simulink subsystem "DYNAMICS"  (R2025b)
settings: Solver=VariableStepAuto  StartTime=0.0  StopTime=10.0  RelTol=1e-3
settings Model: Creator=antoniohernandez-rodiciomateos  LastModifiedBy=antoniohernandez-rodiciomateos

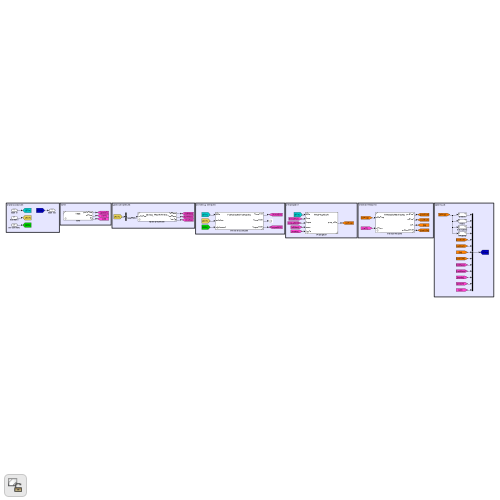
[thumbnail: Simulink's stored preview of the top-level diagram]
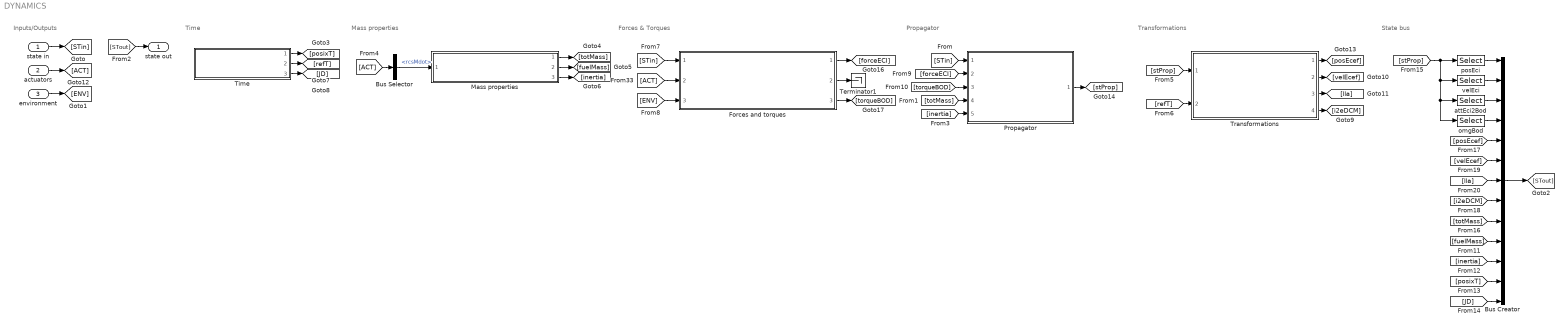
== system DYNAMICS ==
  note: Inputs/Outputs
  note: Mass properties
  note: Time
  note: Forces & Torques
  note: Propagator
  note: Transformations
  note: State bus
  state in : Inport  OutDataTypeStr=Bus: state_bus
  actuators : Inport  Port=2
  environment : Inport  Port=3  OutDataTypeStr=Bus: environment_bus
  Bus Creator : BusCreator  Inputs=13  OutDataTypeStr=Bus: state_bus  NonVirtualBus=on
      settings: InheritFromInputs=off
  Bus Selector : BusSelector  OutputSignals=rcsMdot
  Forces and torques : Subsystem  ReferencedSubsystem=FORCESANDTORQUES  refSurf=simData.aero.refSurf  dc=simData.aero.dragCoeff  rwAllocationMatrix=simData.rw.rwAllocationMatrix  rwInertias=simData.rw.rwInertia  mtqAllocationMatrix=simData.mtq.mtqAllocationMatrix  rcsPositionMatrix=simData.rcs.rcsPositionMatrix  rcsDirectionMatrix=simData.rcs.rcsDirectionMatrix  extPertMag=simData.pert.extPertMag  extPertSeed=simData.pert.pertNoiseSeeds
  Mass properties : Subsystem  ReferencedSubsystem=MASS_PROPERTIES  dryMass=simData.massProperties.dryMass  initFuelMass=simData.ic.initFuelMass  dryInertia=simData.massProperties.dryInertia  fullInertia=simData.massProperties.fullInertia  inertiaBp=simData.massProperties.inertiaBP  inertiaTab=simData.massProperties.inertiaTab
  Propagator : Subsystem  ReferencedSubsystem=PROPAGATOR  quatConv=q4 (scalar last)  forcesFrame=Inertial  r0=simData.ic.r0  v0=simData.ic.v0  att0=simData.ic.att0  omg0=simData.ic.omg0
  Terminator1 : Terminator
  Time : Subsystem  ReferencedSubsystem=TIME  initPosixTime=simData.ic.initTimeUTCPosix  refPosixTime=simData.cts.refTime
  Transformations : Subsystem  ReferencedSubsystem=TRANSFORMATIONS  omgCelBod=simData.cts.omgCelBod
  attEci2Bod : Selector  InputPortWidth=13  IndexOptions=Index vector (dialog)  Indices=[7:10]  OutputSizes=1
  omgBod : Selector  InputPortWidth=13  IndexOptions=Index vector (dialog)  Indices=[11:13]  OutputSizes=1
  posEci : Selector  InputPortWidth=13  IndexOptions=Index vector (dialog)  Indices=[1:3]  OutputSizes=1
  velEci : Selector  InputPortWidth=13  IndexOptions=Index vector (dialog)  Indices=[4:6]  OutputSizes=1
  state out : Outport  OutDataTypeStr=Bus: state_bus
  wires:
  actuators/1 -> [ACT]
  environment/1 -> [ENV]
  state in/1 -> [STin]
  [STin] -> Propagator/1
  Mass properties/3 -> [inertia]
  Mass properties/1 -> [totMass]
  Mass properties/2 -> [fuelMass]
  Bus Selector/1 -> Mass properties/1  "<rcsMdot>"
  [totMass] -> Propagator/4
  Time/3 -> [JD]
  Time/2 -> [refT]
  Time/1 -> [posixT]
  [STout] -> state out/1
  Transformations/3 -> [lla]
  [refT] -> Transformations/2
  Transformations/2 -> [velEcef]
  Transformations/4 -> [i2eDCM]
  [stProp] -> Transformations/1
  Transformations/1 -> [posEcef]
  [inertia] -> Propagator/5
  Propagator/1 -> [stProp]
  [STin] -> Forces and torques/1
  [ACT] -> Forces and torques/2
  [ENV] -> Forces and torques/3
  Forces and torques/1 -> [forceECI]
  Forces and torques/2 -> Terminator1/1
  Forces and torques/3 -> [torqueBOD]
  [forceECI] -> Propagator/2
  [torqueBOD] -> Propagator/3
  [stProp] -> omgBod/1, attEci2Bod/1, velEci/1, posEci/1
  [i2eDCM] -> Bus Creator/8
  Bus Creator/1 -> [STout]
  [JD] -> Bus Creator/13
  [totMass] -> Bus Creator/9
  [fuelMass] -> Bus Creator/10
  omgBod/1 -> Bus Creator/4
  velEci/1 -> Bus Creator/2
  attEci2Bod/1 -> Bus Creator/3
  [inertia] -> Bus Creator/11
  [posixT] -> Bus Creator/12
  posEci/1 -> Bus Creator/1
  [posEcef] -> Bus Creator/5
  [velEcef] -> Bus Creator/6
  [lla] -> Bus Creator/7
  [ACT] -> Bus Selector/1
